simulink model "trifase"  (R2013a)
settings: Solver=ode45  StartTime=0.0  StopTime=2/60  RelTol=1e-3
values from neighbouring files (symbols this model uses):
  R = 50    [sim1.m]
  V_source = 100    [sim1.m]
libraries: powerlib x11, powerlib_meascontrol x4
settings Model: Creator=dello  LastModifiedBy=dello
settings DataIOCC: ExternalInput=[V_source, R]  SignalLoggingName=trifasico
settings OptimizationCC: BlockReduction=off

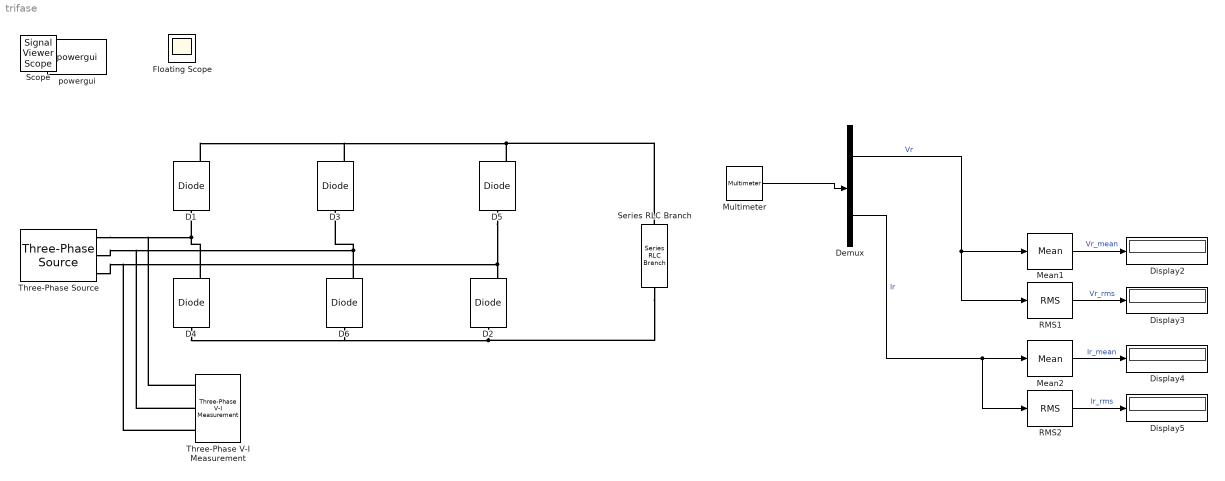
== system trifase ==
  D{1..6} (6 alike) : powerlib/Power Electronics/Diode  Ron=0.001  Lon=0  Vf=0.8  IC=0  UseSnubber=off  Rs=500  Cs=250e-9  Measurements=on
  Demux : Demux  Outputs=2
  Display{2..5} (4 alike) : Display
  Mean1 : powerlib_meascontrol/Measurements/Mean  Freq=60  Vinit=0  Ts=0
  Mean2 : powerlib_meascontrol/Measurements/Mean  Freq=60  Vinit=0  Ts=0
  Multimeter : powerlib/Measurements/Multimeter  PhasorSimulation=off  OutputType=Complex  sel=[1 2]  L=2  Gain=[1 1]  yselected={'Ub: Series RLC Branch','Ib: Series RLC Branch'};  PSBOutputType=1  PSBequivalent=0  AxesSetting=[0,0.1,-100,100]  Display=0  SavedBlockNames=-11
  RMS1 : powerlib_meascontrol/Measurements/RMS  TrueRMS=on  Freq=60  RMSInit=120  Ts=0
  RMS2 : powerlib_meascontrol/Measurements/RMS  TrueRMS=on  Freq=60  RMSInit=120  Ts=0
  Series RLC Branch : powerlib/Elements/Series RLC Branch  LConnTagsString=__new0  RConnTagsString=__new0  BranchType=R  Resistance=R  Inductance=1e-3  SetiL0=off  InitialCurrent=0  Capacitance=1e-6  Setx0=off  InitialVoltage=0  Measurements=Branch voltage and current
  Three-Phase V-I Measurement : powerlib/Measurements/Three-Phase V-I Measurement  VoltageMeasurement=phase-to-ground  SetLabelV=off  LabelV=Vabc  Vpu=off  VpuLL=off  CurrentMeasurement=no  SetLabelI=off  LabelI=Iabc  Ipu=off  Pbase=100e6  Vbase=500e3  OutputType=Complex  PhasorSimulation=off  PSBequivalent=0
  Three-Phase Source : powerlib/Electrical Sources/Three-Phase Source  Voltage=sqrt(3)*V_source/sqrt(2)  PhaseAngle=0  Frequency=60  InternalConnection=Yg  SpecifyImpedance=off  Resistance=0.00001  Inductance=0  ShortCircuitLevel=100e6  BaseVoltage=0  XRratio=7  BusType=swing  Pref=0  Qref=0  Qmin=-inf  Qmax=inf
  powergui : powerlib/powergui  Priority=1  SimulationMode=Continuous  SolverType=Tustin  SampleTime=50e-6  frequency=60  SPID=off  DisableSnubberDevices=off  DisableRonSwitches=off  DisableVfSwitches=off  SwTol=0  Interpol=off  DisplayEquations=off  frequencyindice=60  Pbase=100e6  ErrMax=1e-4  Iterations=50  UnitsV=kV  UnitsW=MW  FunctionMessages=off  echomessages=off  HookPort=off  EnableUseOfTLC=off  x0status=blocks  RestoreLinks=warning  ResistiveCurrentMeasurement=off  Frange=[0:2:500]  Ylog=off  Xlog=on  ShowGrid=off  save=off  variable=ZData  ZoomFFT=off  StartTime=0.0  cycles=1  DisplayStyle=1  fundamental=60  FreqAxis=off  MaxFrequency=1000  frequencyindicesteady=1  RmsSteady=1  display=off  Ts=0  methode=off
  Floating Scope : Scope
      settings: Floating=on  TimeRange=0.03333333333333333
  Scope : SignalViewerScope  IOType=viewer  RefreshTime=0.035000
  wires:
  Multimeter/1 -> Demux/1
  Demux/1 -> RMS1/1, Mean1/1  "Vr"
  Demux/2 -> RMS2/1, Mean2/1  "Ir"
  Mean1/1 -> Display2/1  "Vr_mean"
  RMS1/1 -> Display3/1  "Vr_rms"
  Mean2/1 -> Display4/1  "Ir_mean"
  RMS2/1 -> Display5/1  "Ir_rms"
  connections:
  Series RLC Branch/LConn1 -- D1/RConn1 -- D3/RConn1 -- D5/RConn1
  D2/LConn1 -- D4/LConn1 -- D6/LConn1 -- Series RLC Branch/RConn1
  D5/LConn1 -- Three-Phase V-I Measurement/LConn3 -- Three-Phase Source/RConn3 -- D2/RConn1
  D4/RConn1 -- Three-Phase V-I Measurement/LConn1 -- Three-Phase Source/RConn1 -- D1/LConn1
  D6/RConn1 -- Three-Phase V-I Measurement/LConn2 -- Three-Phase Source/RConn2 -- D3/LConn1
